simulink model "variosmodelos"  (R2016a)
settings: Solver=ode15s  StartTime=0.0  StopTime=tiempo  MaxStep=0.1  RelTol=1e-3
values from neighbouring files (symbols this model uses):
  K11 = K(1,1,i)    [ejecutarparatodoslosmodelos.m]
  K12 = K(1,2,i)    [ejecutarparatodoslosmodelos.m]
  K21 = K(2,1,i)    [ejecutarparatodoslosmodelos.m]
  K22 = K(2,2,i)    [ejecutarparatodoslosmodelos.m]
  Kc11 = Kc11/Fluyben(i)    [ejecutarparatodoslosmodelos.m]
  Kc22 = Kc22/Fluyben(i)    [ejecutarparatodoslosmodelos.m]
  T11 = T(1,1,i)    [ejecutarparatodoslosmodelos.m]
  T12 = T(1,2,i)    [ejecutarparatodoslosmodelos.m]
  T21 = T(2,1,i)    [ejecutarparatodoslosmodelos.m]
  T22 = T(2,2,i)    [ejecutarparatodoslosmodelos.m]
  Ti11 = Ti11*Fluyben(i)    [ejecutarparatodoslosmodelos.m]
  Ti22 = Ti11*Fluyben(i)    [ejecutarparatodoslosmodelos.m]
  tm11 = tm(1,1,i)    [ejecutarparatodoslosmodelos.m]
  tm12 = tm(1,2,i)    [ejecutarparatodoslosmodelos.m]
  tm21 = tm(2,1,i)    [ejecutarparatodoslosmodelos.m]
  tm22 = tm(2,2,i)    [ejecutarparatodoslosmodelos.m]
libraries: simulink x2
settings Model: Creator=JuanRequez  LastModifiedBy=JuanRequez

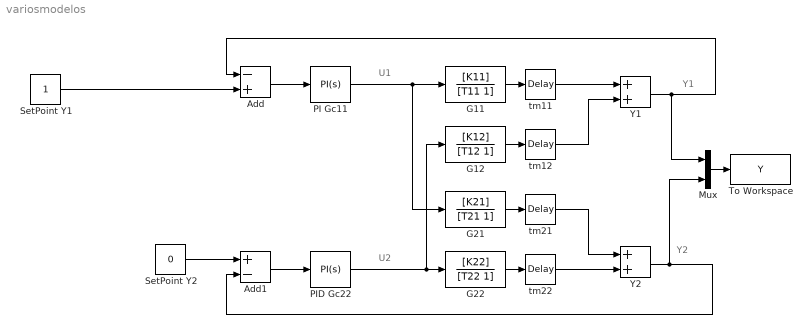
== system variosmodelos ==
  note: Y1
  note: Y2
  note: U2
  note: U1
  Add : Sum  Inputs=-+
  Add1 : Sum  Inputs=+-
  G11 : TransferFcn  Numerator=[K11]  Denominator=[T11 1]
  G12 : TransferFcn  Numerator=[K12]  Denominator=[T12 1]
  G21 : TransferFcn  Numerator=[K21]  Denominator=[T21 1]
  G22 : TransferFcn  Numerator=[K22]  Denominator=[T22 1]
  Mux : Mux  Inputs=2
  PI Gc11 : simulink/Continuous/PID Controller  Controller=PI  TimeDomain=Continuous-time  SampleTime=-1  IntegratorMethod=Forward Euler  FilterMethod=Forward Euler  Form=Ideal  UseFilter=on  ControllerParametersSource=internal  P=Kc11  I=1/Ti11  D=0  N=100  InitialConditionSource=internal  InitialConditionForIntegrator=0  InitialConditionForFilter=0  ExternalReset=none  LimitOutput=off  UpperSaturationLimit=inf  LowerSaturationLimit=-inf  LinearizeAsGain=on  AntiWindupMode=none  Kb=1  TrackingMode=off  Kt=1  PParamMin=[]  PParamMax=[]  IParamMin=[]  IParamMax=[]  DParamMin=[]  DParamMax=[]  NParamMin=[]  NParamMax=[]  KbParamMin=[]  KbParamMax=[]  KtParamMin=[]  KtParamMax=[]  POutMin=[]  POutMax=[]  IOutMin=[]  IOutMax=[]  DOutMin=[]  DOutMax=[]  NOutMin=[]  NOutMax=[]  KbOutMin=[]  KbOutMax=[]  KtOutMin=[]  KtOutMax=[]  IntegratorOutMin=[]  IntegratorOutMax=[]  FilterOutMin=[]  FilterOutMax=[]  SumOutMin=[]  SumOutMax=[]  SumI1OutMin=[]  SumI1OutMax=[]  SumI2OutMin=[]  SumI2OutMax=[]  SumI3OutMin=[]  SumI3OutMax=[]  SumDOutMin=[]  SumDOutMax=[]  SaturationOutMin=[]  SaturationOutMax=[]  IntegratorContinuousStateAttributes=''  IntegratorStateMustResolveToSignalObject=off  IntegratorRTWStateStorageClass=Auto  FilterContinuousStateAttributes=''  FilterStateMustResolveToSignalObject=off  FilterRTWStateStorageClass=Auto  DifferentiatorICPrevScaledInput=0  DifferentiatorOutMin=[]  DifferentiatorOutMax=[]
  PID Gc22 : simulink/Continuous/PID Controller  Controller=PI  TimeDomain=Continuous-time  SampleTime=-1  IntegratorMethod=Forward Euler  FilterMethod=Forward Euler  Form=Ideal  UseFilter=on  ControllerParametersSource=internal  P=Kc22  I=1/Ti22  D=0  N=100  InitialConditionSource=internal  InitialConditionForIntegrator=0  InitialConditionForFilter=0  ExternalReset=none  LimitOutput=off  UpperSaturationLimit=inf  LowerSaturationLimit=-inf  LinearizeAsGain=on  AntiWindupMode=none  Kb=1  TrackingMode=off  Kt=1  PParamMin=[]  PParamMax=[]  IParamMin=[]  IParamMax=[]  DParamMin=[]  DParamMax=[]  NParamMin=[]  NParamMax=[]  KbParamMin=[]  KbParamMax=[]  KtParamMin=[]  KtParamMax=[]  POutMin=[]  POutMax=[]  IOutMin=[]  IOutMax=[]  DOutMin=[]  DOutMax=[]  NOutMin=[]  NOutMax=[]  KbOutMin=[]  KbOutMax=[]  KtOutMin=[]  KtOutMax=[]  IntegratorOutMin=[]  IntegratorOutMax=[]  FilterOutMin=[]  FilterOutMax=[]  SumOutMin=[]  SumOutMax=[]  SumI1OutMin=[]  SumI1OutMax=[]  SumI2OutMin=[]  SumI2OutMax=[]  SumI3OutMin=[]  SumI3OutMax=[]  SumDOutMin=[]  SumDOutMax=[]  SaturationOutMin=[]  SaturationOutMax=[]  IntegratorContinuousStateAttributes=''  IntegratorStateMustResolveToSignalObject=off  IntegratorRTWStateStorageClass=Auto  FilterContinuousStateAttributes=''  FilterStateMustResolveToSignalObject=off  FilterRTWStateStorageClass=Auto  DifferentiatorICPrevScaledInput=0  DifferentiatorOutMin=[]  DifferentiatorOutMax=[]
  SetPoint Y1 : Constant
  SetPoint Y2 : Constant  Value=0
  To Workspace : ToWorkspace  VariableName=Y  SaveFormat=Timeseries  SampleTime=-1
  "Y1 " : Sum
  Y2 : Sum
  tm11 : TransportDelay  DelayTime=tm11
  tm12 : TransportDelay  DelayTime=tm12
  tm21 : TransportDelay  DelayTime=tm21
  tm22 : TransportDelay  DelayTime=tm22
  wires:
  PI Gc11/1 -> G21/1, G11/1
  PID Gc22/1 -> G12/1, G22/1
  Add/1 -> PI Gc11/1
  Add1/1 -> PID Gc22/1
  G11/1 -> tm11/1
  G12/1 -> tm12/1
  G21/1 -> tm21/1
  G22/1 -> tm22/1
  "Y1 "/1 -> Mux/1, Add/1
  Y2/1 -> Mux/2, Add1/2
  tm11/1 -> "Y1 "/1
  tm12/1 -> "Y1 "/2
  tm21/1 -> Y2/1
  tm22/1 -> Y2/2
  SetPoint Y2/1 -> Add1/1
  SetPoint Y1/1 -> Add/2
  Mux/1 -> To Workspace/1
